simulink model "PREPROCESS"  (R2020b)
settings: Solver=FixedStepAuto  StartTime=0.0  StopTime=31622400  FixedStep=60  RelTol=1e-3
libraries: simulink x30
(part 1 of 2)
settings Model: Creator=khfa  LastModifiedBy=khfa

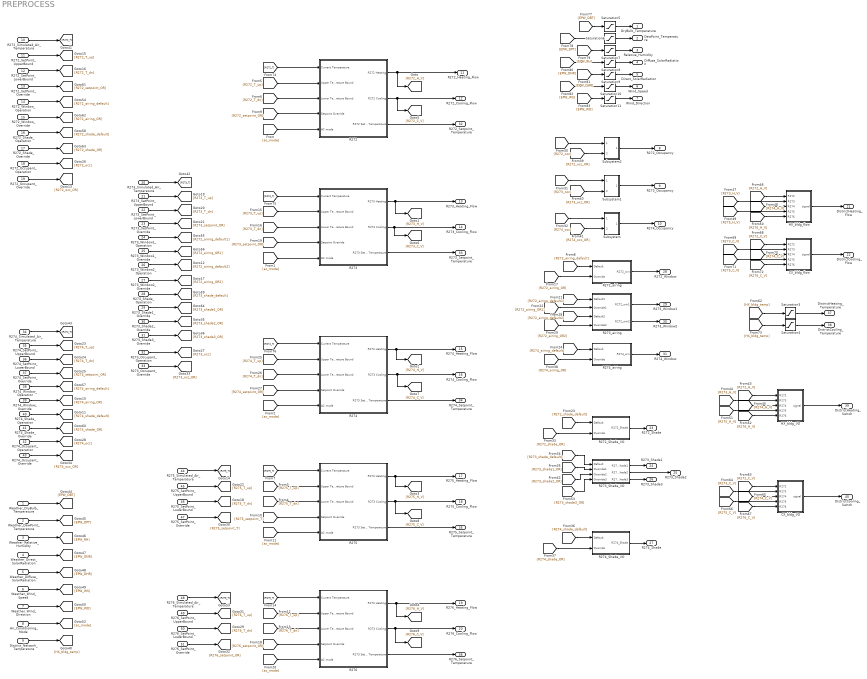
== system PREPROCESS ==
  Weather_DryBulb_Temperature : Inport
  Weather_DewPoint_Temperature : Inport  Port=2
  Weather_Relative_Humidity : Inport  Port=3
  Weather_Direct_SolarRadiation : Inport  Port=4
  Weather_Diffuse_SolarRadiation : Inport  Port=5
  Weather_Wind_Speed : Inport  Port=6
  Weather_Wind_Direction : Inport  Port=7
  Air_Conditioning_Mode : Inport  Port=8
  District_Network_Temperature : Inport  Port=9
  R272_Simulated_Air_Temperature : Inport  Port=10  SampleTime=60
  R272_SetPoint_UpperBound : Inport  Port=11
  R272_SetPoint_LowerBound : Inport  Port=12
  R272_SetPoint_Override : Inport  Port=13
  R272_Window_Operation : Inport  Port=14
  R272_Window_Override : Inport  Port=15
  R272_Shade_Operation : Inport  Port=16
  R272_Shade_Override : Inport  Port=17
  R272_Occupant_Operation : Inport  Port=18
  R272_Occupant_Override : Inport  Port=19
  R273_Simulated_Air_Temperature : Inport  Port=20  SampleTime=60
  R273_SetPoint_UpperBound : Inport  Port=21
  R273_SetPoint_LowerBound : Inport  Port=22
  R273_SetPoint_Override : Inport  Port=23
  R273_Window1_Operation : Inport  Port=24
  R273_Window1_Override : Inport  Port=25
  R273_Window2_Operation : Inport  Port=26
  R273_Window2_Override : Inport  Port=27
  R273_Shade_Operation : Inport  Port=28
  R273_Shade1_Override : Inport  Port=29
  R273_Shade2_Override : Inport  Port=30
  R273_Shade3_Override : Inport  Port=31
  R273_Occupant_Operation : Inport  Port=32
  R273_Occupant_Override : Inport  Port=33
  R274_Simulated_Air_Temperature : Inport  Port=34  SampleTime=60
  R274_SetPoint_UpperBound : Inport  Port=35
  R274_SetPoint_LowerBound : Inport  Port=36
  R274_SetPoint_Override : Inport  Port=37
  R274_Window_Operation : Inport  Port=38
  R274_Window_Override : Inport  Port=39
  R274_Shade_Operation : Inport  Port=40
  R274_Shade_Override : Inport  Port=41
  R274_Occupant_Operation : Inport  Port=42
  R274_Occupant_Override : Inport  Port=43
  R275_Simulated_Air_Temperature : Inport  Port=44  SampleTime=60
  R275_SetPoint_UpperBound : Inport  Port=45
  R275_SetPoint_LowerBound : Inport  Port=46
  R275_SetPoint_Override : Inport  Port=47
  R276_Simulated_Air_Temperature : Inport  Port=48  SampleTime=60
  R276_SetPoint_UpperBound : Inport  Port=49
  R276_SetPoint_LowerBound : Inport  Port=50
  R276_SetPoint_Override : Inport  Port=51
  CX_bldg_I/O : Subsystem
  CX_bldg_flow : Subsystem
  HX_bldg_I/O : Subsystem
  HX_bldg_flow : Subsystem
  R272 : Subsystem
  R272_Shade_I/O : Subsystem
  R272_airing : Subsystem
  R273 : Subsystem
  R273_Shade_I/O : Subsystem
  R273_airing : Subsystem
  R274 : Subsystem
  R274_Shade_I/O : Subsystem
  R274_airing : Subsystem
  R275 : Subsystem
  R276 : Subsystem
  Saturation10 : Saturate  UpperLimit=50  LowerLimit=0
  Saturation11 : Saturate  UpperLimit=360  LowerLimit=0
  Saturation3 : Saturate  UpperLimit=60  LowerLimit=20
  Saturation4 : Saturate  UpperLimit=40  LowerLimit=0
  Saturation5 : Saturate  UpperLimit=60  LowerLimit=-60
  Saturation6 : Saturate  UpperLimit=60  LowerLimit=-60
  Saturation7 : Saturate  UpperLimit=100  LowerLimit=0
  Saturation8 : Saturate  UpperLimit=1000  LowerLimit=0
  Saturation9 : Saturate  UpperLimit=1500  LowerLimit=0
  Subsystem : Subsystem
  Subsystem1 : Subsystem
  Subsystem2 : Subsystem
  DryBulb_Temperature : Outport
  DewPoint_Temperature : Outport  Port=2
  Relative_Humidity : Outport  Port=3
  Diffuse_SolarRadiation : Outport  Port=4
  Direct_SolarRadiation : Outport  Port=5
  Wind_Speed : Outport  Port=6
  Wind_Direction : Outport  Port=7
  R272_Occupancy : Outport  Port=8
  R273_Occupancy : Outport  Port=9
  R274_Occupancy : Outport  Port=10
  R272_Heating_Flow : Outport  Port=11
  R272_Cooling_Flow : Outport  Port=12
  R273_Heating_Flow : Outport  Port=13
  R273_Cooling_Flow : Outport  Port=14
  R274_Heating_Flow : Outport  Port=15
  R274_Cooling_Flow : Outport  Port=16
  R275_Heating_Flow : Outport  Port=17
  R275_Cooling_Flow : Outport  Port=18
  R276_Heating_Flow : Outport  Port=19
  R276_Cooling_Flow : Outport  Port=20
  DistrictHeating_Flow : Outport  Port=21
  DistrictCooling_Flow : Outport  Port=22
  R272_Shade : Outport  Port=23
  R273_Shade1 : Outport  Port=24
  R273_Shade2 : Outport  Port=25
  R273_Shade3 : Outport  Port=26
  R274_Shade : Outport  Port=27
  R272_Window : Outport  Port=28
  R273_Window1 : Outport  Port=29
  R273_Window2 : Outport  Port=30
  R274_Window : Outport  Port=31
  R272_Setpoint_Temperature : Outport  Port=32
  R273_Setpoint_Temperature : Outport  Port=33
  R274_Setpoint_Temperature : Outport  Port=34
  R275_Setpoint_Temperature : Outport  Port=35
  R276_Setpoint_Temperature : Outport  Port=36
  DistrictHeating_Temperature : Outport  Port=37
  DistrictCooling_Temperature : Outport  Port=38
  DistrictHeating_Switch : Outport  Port=39
  DistrictCooling_Switch : Outport  Port=40
  wires:
  Saturation11/1 -> Wind_Direction/1
  Saturation6/1 -> DewPoint_Temperature/1
  Saturation7/1 -> Relative_Humidity/1
  Saturation8/1 -> Diffuse_SolarRadiation/1
  Saturation10/1 -> Wind_Speed/1
  R272_Shade_I/O/1(R272_Shade) -> R272_Shade/1
  R273_Shade_I/O/1(R273_Shade1) -> R273_Shade1/1
  R275_Simulated_Air_Temperature/1 -> [R275_T]
  R275_SetPoint_Override/1 -> [R275_setpoint_T]
  R275_SetPoint_LowerBound/1 -> [R275_T_dn]
  R274/3(R273 Setpoint Temperature) -> R274_Setpoint_Temperature/1
  R275/3(R273 Setpoint Temperature) -> R275_Setpoint_Temperature/1
  R273_Window2_Operation/1 -> [R272_airing_default2]
  District_Network_Temperature/1 -> [HX_bldg_temp]
  Weather_Direct_SolarRadiation/1 -> [EPW_DNR]
  R273/3(R273 Setpoint Temperature) -> R273_Setpoint_Temperature/1
  Weather_Wind_Speed/1 -> [EPW_WS]
  R273_Occupant_Operation/1 -> [R273_occ]
  R273_SetPoint_LowerBound/1 -> [R273_T_dn]
  R273_Simulated_Air_Temperature/1 -> [R273_T]
  R273_SetPoint_Override/1 -> [R273_setpoint_OR]
  Air_Conditioning_Mode/1 -> [ac_mode]
  R273_Window1_Operation/1 -> [R272_airing_default1]
  R273_SetPoint_UpperBound/1 -> [R273_T_up]
  R273_Shade_Operation/1 -> [R273_shade_default]
  R273_Window1_Override/1 -> [R272_airing_OR1]
  R273_Shade1_Override/1 -> [R273_shade1_OR]
  R273_Window2_Override/1 -> [R272_airing_OR2]
  Weather_Relative_Humidity/1 -> [EPW_RH]
  Weather_Diffuse_SolarRadiation/1 -> [EPW_DHR]
  Weather_Wind_Direction/1 -> [EPW_WD]
  CX_bldg_I/O/1(signal) -> DistrictCooling_Switch/1
  Saturation4/1 -> DistrictCooling_Temperature/1
  HX_bldg_I/O/1(signal) -> DistrictHeating_Switch/1
  Saturation3/1 -> DistrictHeating_Temperature/1
  R272_SetPoint_UpperBound/1 -> [R272_T_up]
  R272_Window_Operation/1 -> [R272_airing_default]
  R272_Occupant_Operation/1 -> [R272_occ]
  R272_Shade_Operation/1 -> [R272_shade_default]
  R272_Window_Override/1 -> [R272_airing_OR]
  R272_SetPoint_Override/1 -> [R272_setpoint_OR]
  [R276_C_V] -> CX_bldg_I/O/5(R276)
  [R275_C_V] -> CX_bldg_flow/4(R275)
  [R272_H_V] -> HX_bldg_I/O/1(R272)
  R272_SetPoint_LowerBound/1 -> [R272_T_dn]
  [R272_setpoint_OR] -> R272/4(Setpoint Override)
  Saturation5/1 -> DryBulb_Temperature/1
  [R272_T] -> R272/1(Current Temperature)
  [R274_C_V] -> CX_bldg_I/O/3(R274)
  [R275_H_V] -> HX_bldg_I/O/4(R275)
  R272/3(R272 Setpoint Temperature) -> R272_Setpoint_Temperature/1
  [R273_H_V] -> HX_bldg_I/O/2(R273)
  [R276_H_V] -> HX_bldg_I/O/5(R276)
  [R272_H_V] -> HX_bldg_flow/1(R272)
  [R276_T_up] -> R276/2(Upper Temperature Bound)
  [R273_T_up] -> R273/2(Upper Temperature Bound)
  [R275_T_up] -> R275/2(Upper Temperature Bound)
  Saturation9/1 -> Direct_SolarRadiation/1
  [EPW_DPT] -> Saturation6/1
  [R272_airing_default] -> R272_airing/1(Default)
  R273/2(R273 Cooling) -> R273_Cooling_Flow/1, [R273_C_V]
  R272/1(R272 Heating) -> R272_Heating_Flow/1, [R272_H_V]
  R274/1(R273 Heating) -> R274_Heating_Flow/1, [R274_H_V]
  R275/1(R273 Heating) -> R275_Heating_Flow/1, [R275_H_V]
  [R275_T] -> R275/1(Current Temperature)
  [R273_setpoint_OR] -> R273/4(Setpoint Override)
  [R276_C_V] -> CX_bldg_flow/5(R276)
  R272_Simulated_Air_Temperature/1 -> [R272_T]
  [R273_C_V] -> CX_bldg_flow/2(R273)
  [EPW_DHR] -> Saturation9/1
  [R274_T_dn] -> R274/3(Lower Temperature Bound)
  R272/2(R272 Cooling) -> R272_Cooling_Flow/1, [R272_C_V]
  R272_Shade_Override/1 -> [R272_shade_OR]
  [R273_T_dn] -> R273/3(Lower Temperature Bound)
  R273/1(R273 Heating) -> [R273_H_V], R273_Heating_Flow/1
  [EPW_RH] -> Saturation7/1
  [ac_mode] -> R272/5(AC mode)
  [EPW_DBT] -> Saturation5/1
  [R274_T_up] -> R274/2(Upper Temperature Bound)
  [R272_C_V] -> CX_bldg_I/O/1(R272)
  [HX_bldg_temp] -> Saturation3/1
  [R274_shade_OR] -> R274_Shade_I/O/2(Override)
  Weather_DewPoint_Temperature/1 -> [EPW_DPT]
  [HX_bldg_temp] -> Saturation4/1
  [R273_shade1_OR] -> R273_Shade_I/O/2(Override1)
  [R273_shade_default] -> R273_Shade_I/O/1(Default)
  [R274_H_V] -> HX_bldg_I/O/3(R274)
  R276_SetPoint_LowerBound/1 -> [R276_T_dn]
  R276_Simulated_Air_Temperature/1 -> [R276_T]
  CX_bldg_flow/1(signal) -> DistrictCooling_Flow/1
  [R272_airing_default1] -> R273_airing/1(Default1)
  R276/1(R273 Heating) -> R276_Heating_Flow/1, [R276_H_V]
  R274_SetPoint_UpperBound/1 -> [R274_T_up]
  R274_SetPoint_LowerBound/1 -> [R274_T_dn]
  R276_SetPoint_Override/1 -> [R276_setpoint_OR]
  [EPW_WD] -> Saturation11/1
  [R274_airing_OR] -> R274_airing/2(Override)
  HX_bldg_flow/1(signal) -> DistrictHeating_Flow/1
  [R273_T] -> R273/1(Current Temperature)
  [R272_airing_default2] -> R273_airing/3(Default2)
  [R272_shade_OR] -> R272_Shade_I/O/2(Override)
  [R272_airing_OR2] -> R273_airing/4(Override2)
  R274_Shade_Override/1 -> [R274_shade_OR]
  [R272_airing_OR1] -> R273_airing/2(Override1)
  [R272_shade_default] -> R272_Shade_I/O/1(Default)
  [R274_H_V] -> HX_bldg_flow/3(R274)
  [R272_C_V] -> CX_bldg_flow/1(R272)
  R275_SetPoint_UpperBound/1 -> [R275_T_up]
  R276/2(R273 Cooling) -> R276_Cooling_Flow/1, [R276_C_V]
  [EPW_WS] -> Saturation10/1
  [R274_C_V] -> CX_bldg_flow/3(R274)
  [R273_C_V] -> CX_bldg_I/O/2(R273)
  [R275_T_dn] -> R275/3(Lower Temperature Bound)
  [ac_mode] -> R275/5(AC mode)
  [R272_T_dn] -> R272/3(Lower Temperature Bound)
  R274_Window_Operation/1 -> [R274_airing_default]
  [R276_setpoint_OR] -> R276/4(Setpoint Override)
  [R275_setpoint_T] -> R275/4(Setpoint Override)
  [R275_C_V] -> CX_bldg_I/O/4(R275)
  [R272_airing_OR] -> R272_airing/2(Override)
  R274_Simulated_Air_Temperature/1 -> [R274_T]
  R274/2(R273 Cooling) -> R274_Cooling_Flow/1, [R274_C_V]
  [R275_H_V] -> HX_bldg_flow/4(R275)
  R276_SetPoint_UpperBound/1 -> [R276_T_up]
  [R274_shade_default] -> R274_Shade_I/O/1(Default)
  [R274_T] -> R274/1(Current Temperature)
  R275/2(R273 Cooling) -> [R275_C_V], R275_Cooling_Flow/1
  R274_Shade_Operation/1 -> [R274_shade_default]
  [R272_T_up] -> R272/2(Upper Temperature Bound)
  R274_Shade_I/O/1(R274_Shade) -> R274_Shade/1
  [ac_mode] -> R276/5(AC mode)
  [R274_airing_default] -> R274_airing/1(Default)
  R274_Window_Override/1 -> [R274_airing_OR]
  [ac_mode] -> R273/5(AC mode)
  Weather_DryBulb_Temperature/1 -> [EPW_DBT]
  [R276_T_dn] -> R276/3(Lower Temperature Bound)
  R273_airing/1(R272_win1) -> R273_Window1/1
  [EPW_DNR] -> Saturation8/1
  R274_SetPoint_Override/1 -> [R274_setpoint_OR]
  R272_airing/1(R272_win) -> R272_Window/1
  R274_airing/1(R274_win) -> R274_Window/1
  [R273_H_V] -> HX_bldg_flow/2(R273)
  [R274_setpoint_OR] -> R274/4(Setpoint Override)
  [R276_T] -> R276/1(Current Temperature)
  R274_Occupant_Operation/1 -> [R274_occ]
  R273_airing/2(R272_win2) -> R273_Window2/1
  R276/3(R273 Setpoint Temperature) -> R276_Setpoint_Temperature/1
  [R276_H_V] -> HX_bldg_flow/5(R276)
  [ac_mode] -> R274/5(AC mode)
  R272_Occupant_Override/1 -> [R272_occ_OR]
  R273_Occupant_Override/1 -> [R273_occ_OR]
  R274_Occupant_Override/1 -> [R274_occ_OR]
  [R274_occ] -> Subsystem/1(In1)
  [R274_occ_OR] -> Subsystem/2(In2)
  Subsystem/1(Out1) -> R274_Occupancy/1
  [R273_occ] -> Subsystem1/1(In1)
  [R273_occ_OR] -> Subsystem1/2(In2)
  Subsystem1/1(Out1) -> R273_Occupancy/1
  [R272_occ] -> Subsystem2/1(In1)
  [R272_occ_OR] -> Subsystem2/2(In2)
  Subsystem2/1(Out1) -> R272_Occupancy/1
  R273_Shade2_Override/1 -> [R273_shade2_OR]
  R273_Shade3_Override/1 -> [R273_shade3_OR]
  R273_Shade_I/O/2(R273_Shade2) -> R273_Shade2/1
  R273_Shade_I/O/3(R273_Shade3) -> R273_Shade3/1
  [R273_shade2_OR] -> R273_Shade_I/O/3(Override2)
  [R273_shade3_OR] -> R273_Shade_I/O/4(Override3)

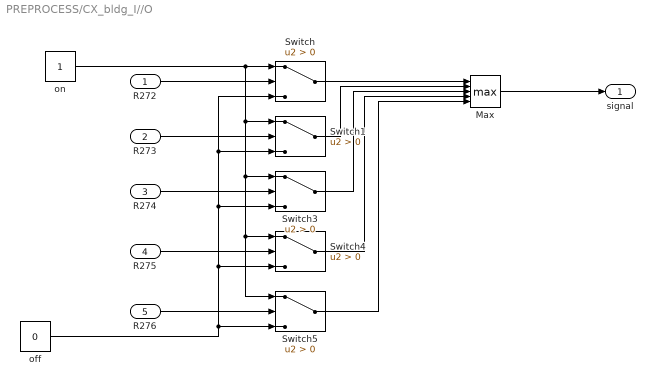
== system PREPROCESS/CX_bldg_I//O ==
  R272 : Inport
  R273 : Inport  Port=2
  R274 : Inport  Port=3
  R275 : Inport  Port=4
  R276 : Inport  Port=5
  Max : MinMax  Function=max  Inputs=5
  Switch{,1,3..5} (5 alike) : Switch  Criteria=u2 > Threshold
  off : Constant  Value=0
  on : Constant
  signal : Outport
  wires:
  on/1 -> Switch5/1, Switch4/1, Switch3/1, Switch1/1, Switch/1
  R272/1 -> Switch/2
  off/1 -> Switch5/3, Switch3/3, Switch1/3, Switch/3, Switch4/3
  R273/1 -> Switch1/2
  R274/1 -> Switch3/2
  Switch/1 -> Max/1
  Switch1/1 -> Max/2
  Switch3/1 -> Max/3
  R276/1 -> Switch5/2
  R275/1 -> Switch4/2
  Switch4/1 -> Max/4
  Switch5/1 -> Max/5
  Max/1 -> signal/1

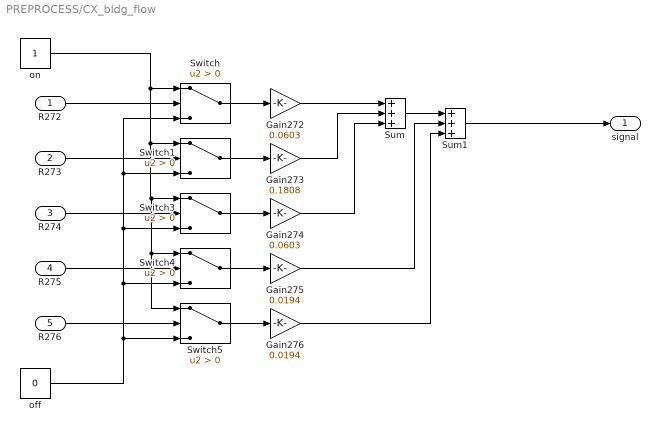
== system PREPROCESS/CX_bldg_flow ==
  R272 : Inport
  R273 : Inport  Port=2
  R274 : Inport  Port=3
  R275 : Inport  Port=4
  R276 : Inport  Port=5
  Gain272 : Gain  Gain=0.0603
  Gain273 : Gain  Gain=0.1808
  Gain274 : Gain  Gain=0.0603
  Gain275 : Gain  Gain=0.0194
  Gain276 : Gain  Gain=0.0194
  Sum : Sum  Inputs=+++
  Sum1 : Sum  Inputs=+++
  Switch{,1,3..5} (5 alike) : Switch  Criteria=u2 > Threshold
  off : Constant  Value=0
  on : Constant
  signal : Outport
  wires:
  Sum/1 -> Sum1/1
  on/1 -> Switch5/1, Switch4/1, Switch3/1, Switch1/1, Switch/1
  R272/1 -> Switch/2
  off/1 -> Switch4/3, Switch3/3, Switch1/3, Switch/3, Switch5/3
  R273/1 -> Switch1/2
  R274/1 -> Switch3/2
  Switch/1 -> Gain272/1
  Switch1/1 -> Gain273/1
  Switch3/1 -> Gain274/1
  Gain272/1 -> Sum/1
  Gain274/1 -> Sum/3
  Gain273/1 -> Sum/2
  Switch4/1 -> Gain275/1
  Gain275/1 -> Sum1/2
  Switch5/1 -> Gain276/1
  R275/1 -> Switch4/2
  R276/1 -> Switch5/2
  Gain276/1 -> Sum1/3
  Sum1/1 -> signal/1

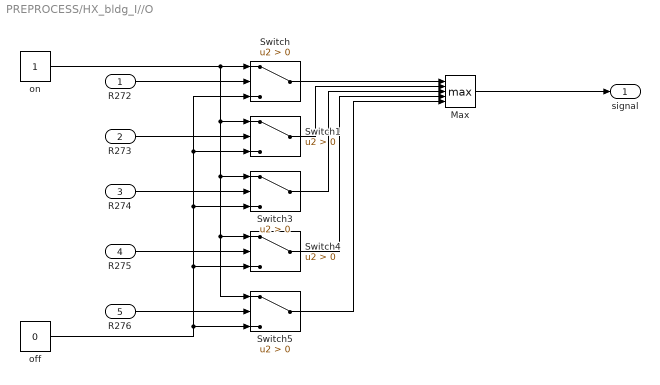
== system PREPROCESS/HX_bldg_I//O ==
  R272 : Inport
  R273 : Inport  Port=2
  R274 : Inport  Port=3
  R275 : Inport  Port=4
  R276 : Inport  Port=5
  Max : MinMax  Function=max  Inputs=5
  Switch{,1,3..5} (5 alike) : Switch  Criteria=u2 > Threshold
  off : Constant  Value=0
  on : Constant
  signal : Outport
  wires:
  Max/1 -> signal/1
  on/1 -> Switch5/1, Switch4/1, Switch3/1, Switch1/1, Switch/1
  R272/1 -> Switch/2
  off/1 -> Switch5/3, Switch3/3, Switch1/3, Switch/3, Switch4/3
  R273/1 -> Switch1/2
  R274/1 -> Switch3/2
  Switch/1 -> Max/1
  Switch1/1 -> Max/2
  Switch3/1 -> Max/3
  R276/1 -> Switch5/2
  R275/1 -> Switch4/2
  Switch4/1 -> Max/4
  Switch5/1 -> Max/5

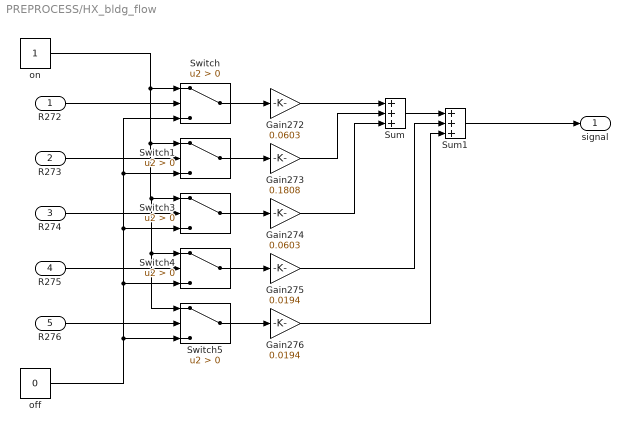
== system PREPROCESS/HX_bldg_flow ==
  R272 : Inport
  R273 : Inport  Port=2
  R274 : Inport  Port=3
  R275 : Inport  Port=4
  R276 : Inport  Port=5
  Gain272 : Gain  Gain=0.0603
  Gain273 : Gain  Gain=0.1808
  Gain274 : Gain  Gain=0.0603
  Gain275 : Gain  Gain=0.0194
  Gain276 : Gain  Gain=0.0194
  Sum : Sum  Inputs=+++
  Sum1 : Sum  Inputs=+++
  Switch{,1,3..5} (5 alike) : Switch  Criteria=u2 > Threshold
  off : Constant  Value=0
  on : Constant
  signal : Outport
  wires:
  Sum/1 -> Sum1/1
  on/1 -> Switch5/1, Switch4/1, Switch3/1, Switch1/1, Switch/1
  R272/1 -> Switch/2
  off/1 -> Switch4/3, Switch3/3, Switch1/3, Switch/3, Switch5/3
  R273/1 -> Switch1/2
  R274/1 -> Switch3/2
  Switch/1 -> Gain272/1
  Switch1/1 -> Gain273/1
  Switch3/1 -> Gain274/1
  Gain272/1 -> Sum/1
  Gain274/1 -> Sum/3
  Gain273/1 -> Sum/2
  Switch4/1 -> Gain275/1
  Gain275/1 -> Sum1/2
  Switch5/1 -> Gain276/1
  R275/1 -> Switch4/2
  R276/1 -> Switch5/2
  Gain276/1 -> Sum1/3
  Sum1/1 -> signal/1

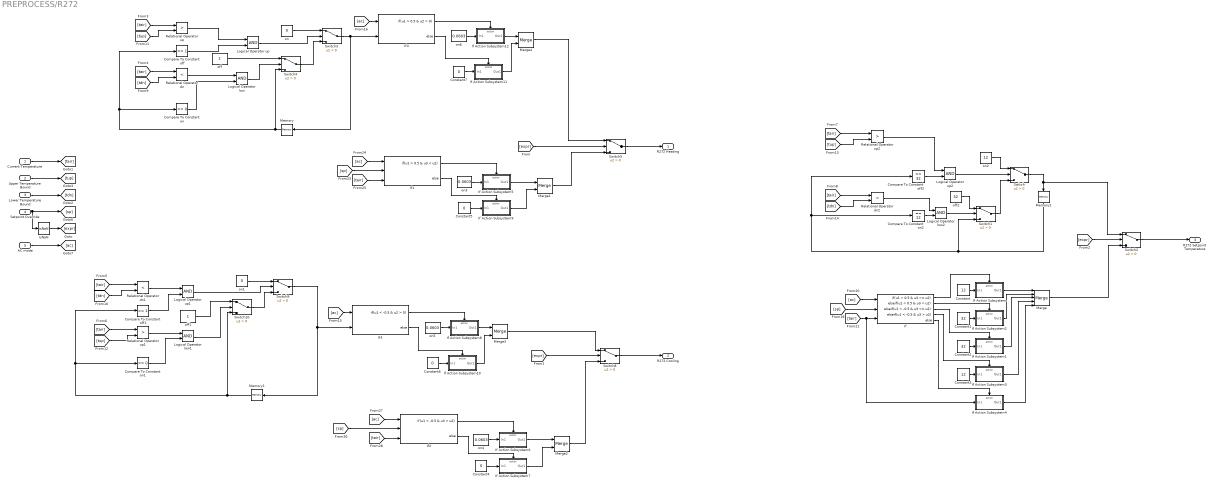
== system PREPROCESS/R272 ==
  Current Temperature : Inport
  Upper Temperature Bound : Inport  Port=2
  Lower Temperature Bound : Inport  Port=3
  Setpoint Override : Inport  Port=4
  AC mode : Inport  Port=5
  Compare To Constant off : simulink/Logic and Bit Operations/Compare To Constant  relop===  const=1  OutDataTypeStr=boolean
  Compare To Constant off1 : simulink/Logic and Bit Operations/Compare To Constant  relop===  const=1  OutDataTypeStr=boolean
  Compare To Constant off2 : simulink/Logic and Bit Operations/Compare To Constant  relop===  const=32  OutDataTypeStr=boolean
  Compare To Constant on : simulink/Logic and Bit Operations/Compare To Constant  relop===  const=0  OutDataTypeStr=boolean
  Compare To Constant on1 : simulink/Logic and Bit Operations/Compare To Constant  relop===  const=0  OutDataTypeStr=boolean
  Compare To Constant on2 : simulink/Logic and Bit Operations/Compare To Constant  relop===  const=12  OutDataTypeStr=boolean
  Constant : Constant  Value=12
  Constant1 : Constant  Value=32
  Constant2 : Constant  Value=32
  Constant3 : Constant  Value=12
  Constant{4..7} (4 alike) : Constant  Value=0
  If : If  NumInputs=3  IfExpression=u1 > 0.5 & u3 >= u2  ElseIfExpressions=u1 > 0.5 & u3 < u2, u1 < -0.5 & u3 <= u2, u1 < -0.5 & u3 > u2
  If Action Subsystem : Subsystem  TreatAsAtomicUnit=on
  If Action Subsystem1 : Subsystem  TreatAsAtomicUnit=on
  If Action Subsystem10 : Subsystem  TreatAsAtomicUnit=on
  If Action Subsystem11 : Subsystem  TreatAsAtomicUnit=on
  If Action Subsystem12 : Subsystem  TreatAsAtomicUnit=on
  If Action Subsystem2 : Subsystem  TreatAsAtomicUnit=on
  If Action Subsystem3 : Subsystem  TreatAsAtomicUnit=on
  If Action Subsystem4 : Subsystem  TreatAsAtomicUnit=on
  If Action Subsystem5 : Subsystem  TreatAsAtomicUnit=on
  If Action Subsystem6 : Subsystem  TreatAsAtomicUnit=on
  If Action Subsystem7 : Subsystem  TreatAsAtomicUnit=on
  If Action Subsystem8 : Subsystem  TreatAsAtomicUnit=on
  If Action Subsystem9 : Subsystem  TreatAsAtomicUnit=on
  If1 : If  NumInputs=3  IfExpression=u1 > 0.5 & u3 < u2
  If2 : If  NumInputs=3  IfExpression=u1 < -0.5 & u3 > u2
  If3 : If  NumInputs=2  IfExpression=u1 < -0.5 & u2 > 0
  If4 : If  NumInputs=2  IfExpression=u1 > 0.5 & u2 > 0
  IsNaN : RelationalOperator  Operator=isNaN  OutDataTypeStr=boolean  RndMeth=Simplest
  Logical Operator low : Logic  AllPortsSameDT=off  OutDataTypeStr=boolean
  Logical Operator low1 : Logic  AllPortsSameDT=off  OutDataTypeStr=boolean
  Logical Operator low2 : Logic  AllPortsSameDT=off  OutDataTypeStr=boolean
  Logical Operator up : Logic  AllPortsSameDT=off  OutDataTypeStr=boolean
  Logical Operator up1 : Logic  AllPortsSameDT=off  OutDataTypeStr=boolean
  Logical Operator up2 : Logic  AllPortsSameDT=off  OutDataTypeStr=boolean
  Memory : Memory
  Memory1 : Memory
  Memory2 : Memory  InitialCondition=12
  Merge : Merge  Inputs=5
  Merge{1..4} (4 alike) : Merge
  Relational Operator dn : RelationalOperator  Operator=<  OutDataTypeStr=boolean  RndMeth=Simplest
  Relational Operator dn1 : RelationalOperator  Operator=<  OutDataTypeStr=boolean  RndMeth=Simplest
  Relational Operator dn2 : RelationalOperator  Operator=<  OutDataTypeStr=boolean  RndMeth=Simplest
  Relational Operator up : RelationalOperator  Operator=>  OutDataTypeStr=boolean  RndMeth=Simplest
  Relational Operator up1 : RelationalOperator  Operator=>  OutDataTypeStr=boolean  RndMeth=Simplest
  Relational Operator up2 : RelationalOperator  Operator=>  OutDataTypeStr=boolean  RndMeth=Simplest
  Switch{,1..5,8..10} (9 alike) : Switch  Criteria=u2 > Threshold
  off : Constant
  off1 : Constant
  off2 : Constant  Value=32
  on : Constant  Value=0
  on1 : Constant  Value=0
  on2 : Constant  Value=12
  on{3..6} (4 alike) : Constant  Value=0.0603
  R272 Heating : Outport
  R272 Cooling : Outport  Port=2
  R272 Setpoint Temperature : Outport  Port=3
  wires:
  [tup] -> Relational Operator up2/2
  [tdn] -> Relational Operator dn2/2
  If4/1 -> If Action Subsystem12/Action
  If4/2 -> If Action Subsystem11/Action
  IsNaN/1 -> [expr]
  If Action Subsystem11/1(Out1) -> Merge4/2
  If/4 -> If Action Subsystem3/Action
  on2/1 -> Switch/1
  [tair] -> If1/3
  If Action Subsystem10/1(Out1) -> Merge3/2
  on6/1 -> If Action Subsystem12/1(In1)
  Merge2/1 -> Switch8/3
  Constant7/1 -> If Action Subsystem11/1(In1)
  [expr] -> Switch5/2
  If1/2 -> If Action Subsystem9/Action
  [sp] -> If/2
  [tup] -> Relational Operator up/2
  Relational Operator dn/1 -> Logical Operator low/1
  [tair] -> If Action Subsystem4/1(In1), If/3
  If Action Subsystem3/1(Out1) -> Merge/4
  If2/1 -> If Action Subsystem6/Action
  If3/1 -> If Action Subsystem8/Action
  If1/1 -> If Action Subsystem5/Action
  [ac] -> If3/1
  Merge4/1 -> Switch5/1
  If2/2 -> If Action Subsystem7/Action
  Compare To Constant off/1 -> Logical Operator up/2
  If Action Subsystem4/1(Out1) -> Merge/5
  Constant2/1 -> If Action Subsystem1/1(In1)
  Lower Temperature Bound/1 -> [tdn]
  Constant6/1 -> If Action Subsystem10/1(In1)
  Relational Operator up2/1 -> Logical Operator up2/1
  on5/1 -> If Action Subsystem8/1(In1)
  Compare To Constant on/1 -> Logical Operator low/2
  Switch5/1 -> R272 Heating/1
  If3/2 -> If Action Subsystem10/Action
  Switch9/1 -> If3/2, Memory1/1
  Switch4/1 -> Switch3/3
  [sp] -> If2/2
  [ac] -> If4/1
  If/5 -> If Action Subsystem4/Action
  on4/1 -> If Action Subsystem6/1(In1)
  Switch8/1 -> R272 Cooling/1
  If Action Subsystem8/1(Out1) -> Merge3/1
  [sp] -> If1/2
  Constant4/1 -> If Action Subsystem7/1(In1)
  Memory/1 -> Compare To Constant on/1, Compare To Constant off/1, Switch4/3
  If Action Subsystem7/1(Out1) -> Merge2/2
  If Action Subsystem6/1(Out1) -> Merge2/1
  Merge3/1 -> Switch8/1
  Logical Operator up/1 -> Switch3/2
  AC mode/1 -> [ac]
  Constant1/1 -> If Action Subsystem2/1(In1)
  Switch3/1 -> Memory/1, If4/2
  [tair] -> If2/3
  If Action Subsystem1/1(Out1) -> Merge/3
  If Action Subsystem5/1(Out1) -> Merge1/1
  If Action Subsystem/1(Out1) -> Merge/1
  If Action Subsystem9/1(Out1) -> Merge1/2
  Merge1/1 -> Switch5/3
  on3/1 -> If Action Subsystem5/1(In1)
  If/2 -> If Action Subsystem2/Action
  Setpoint Override/1 -> IsNaN/1, [sp]
  [ac] -> If2/1
  off1/1 -> Switch10/1
  [tair] -> Relational Operator up2/1
  If/3 -> If Action Subsystem1/Action
  Logical Operator low1/1 -> Switch10/2
  Compare To Constant on1/1 -> Logical Operator low1/2
  Compare To Constant off2/1 -> Logical Operator up2/2
  [tair] -> Relational Operator dn2/1
  [tair] -> Relational Operator up1/1
  [tair] -> Relational Operator dn1/1
  If/1 -> If Action Subsystem/Action
  Constant/1 -> If Action Subsystem/1(In1)
  Logical Operator up2/1 -> Switch/2
  Constant3/1 -> If Action Subsystem3/1(In1)
  Logical Operator low2/1 -> Switch1/2
  Compare To Constant on2/1 -> Logical Operator low2/2
  Memory2/1 -> Compare To Constant on2/1, Compare To Constant off2/1, Switch1/3
  off2/1 -> Switch1/1
  Switch1/1 -> Switch/3
  Switch2/1 -> R272 Setpoint Temperature/1
  [ac] -> If1/1
  [tair] -> Relational Operator dn/1
  [expr] -> Switch8/2
  [tair] -> Relational Operator up/1
  If Action Subsystem12/1(Out1) -> Merge4/1
  Relational Operator dn2/1 -> Logical Operator low2/1
  Logical Operator low/1 -> Switch4/2
  Upper Temperature Bound/1 -> [tup]
  Compare To Constant off1/1 -> Logical Operator up1/2
  Merge/1 -> Switch2/3
  Memory1/1 -> Compare To Constant on1/1, Compare To Constant off1/1, Switch10/3
  [tup] -> Relational Operator up1/2
  [tdn] -> Relational Operator dn1/2
  Relational Operator up1/1 -> Logical Operator low1/1
  Relational Operator dn1/1 -> Logical Operator up1/1
  off/1 -> Switch4/1
  [ac] -> If/1
  Switch10/1 -> Switch9/3
  [tdn] -> Relational Operator dn/2
  Constant5/1 -> If Action Subsystem9/1(In1)
  Relational Operator up/1 -> Logical Operator up/1
  on/1 -> Switch3/1
  [expr] -> Switch2/2
  If Action Subsystem2/1(Out1) -> Merge/2
  Logical Operator up1/1 -> Switch9/2
  Current Temperature/1 -> [tair]
  Switch/1 -> Switch2/1, Memory2/1
  on1/1 -> Switch9/1

== system PREPROCESS/R272_Shade_I//O ==
  Default : Inport
  Override : Inport  Port=2
  Constant : Constant
  Constant1 : Constant  Value=0
  IsNaN : RelationalOperator  Operator=isNaN  OutDataTypeStr=boolean  RndMeth=Simplest
  R272_lum_limit : Switch  Criteria=u2 > Threshold  Threshold=50
  Switch : Switch  Criteria=u2 > Threshold
  Switch1 : Switch  Criteria=u2 > Threshold
  off1 : Constant
  on1 : Constant  Value=0
  R272_Shade : Outport
  wires:
  off1/1 -> R272_lum_limit/3
  on1/1 -> R272_lum_limit/1
  Default/1 -> R272_lum_limit/2
  Constant/1 -> Switch/1
  Constant1/1 -> Switch/3
  Override/1 -> IsNaN/1, Switch/2
  R272_lum_limit/1 -> Switch1/1
  Switch1/1 -> R272_Shade/1
  Switch/1 -> Switch1/3
  IsNaN/1 -> Switch1/2

== system PREPROCESS/R272_airing ==
  Default : Inport
  Override : Inport  Port=2
  Constant : Constant  Value=-49
  Constant1 : Constant  Value=99
  IsNaN : RelationalOperator  Operator=isNaN  OutDataTypeStr=boolean  RndMeth=Simplest
  Switch : Switch  Criteria=u2 > Threshold
  Switch1 : Switch  Criteria=u2 > Threshold
  R272_win : Outport
  wires:
  Constant/1 -> Switch/1
  Constant1/1 -> Switch/3
  Override/1 -> IsNaN/1, Switch/2
  Switch/1 -> Switch1/3
  Switch1/1 -> R272_win/1
  Default/1 -> Switch1/1
  IsNaN/1 -> Switch1/2

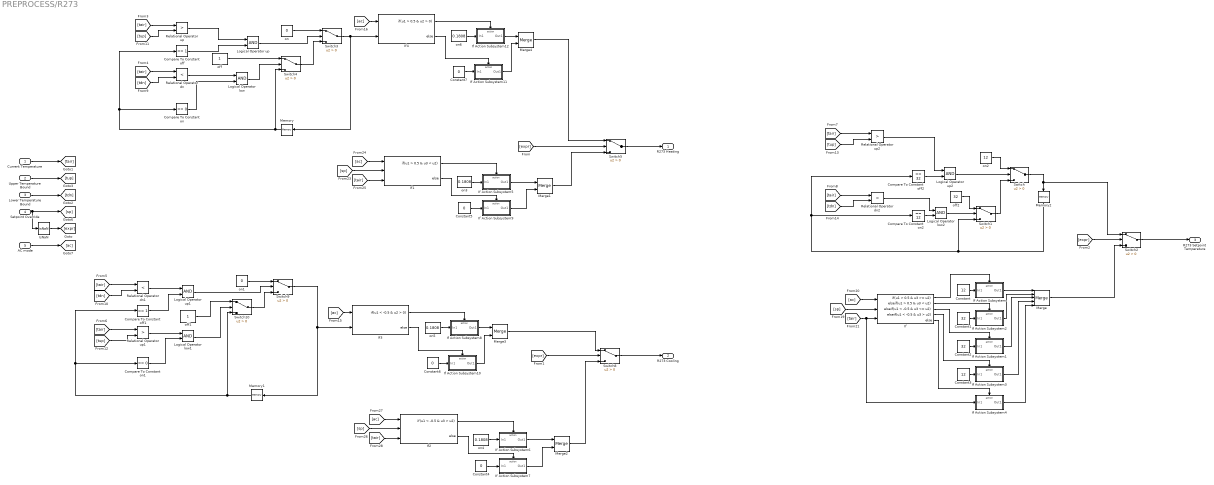
== system PREPROCESS/R273 ==
  Current Temperature : Inport
  Upper Temperature Bound : Inport  Port=2
  Lower Temperature Bound : Inport  Port=3
  Setpoint Override : Inport  Port=4
  AC mode : Inport  Port=5
  Compare To Constant off : simulink/Logic and Bit Operations/Compare To Constant  relop===  const=1  OutDataTypeStr=boolean
  Compare To Constant off1 : simulink/Logic and Bit Operations/Compare To Constant  relop===  const=1  OutDataTypeStr=boolean
  Compare To Constant off2 : simulink/Logic and Bit Operations/Compare To Constant  relop===  const=32  OutDataTypeStr=boolean
  Compare To Constant on : simulink/Logic and Bit Operations/Compare To Constant  relop===  const=0  OutDataTypeStr=boolean
  Compare To Constant on1 : simulink/Logic and Bit Operations/Compare To Constant  relop===  const=0  OutDataTypeStr=boolean
  Compare To Constant on2 : simulink/Logic and Bit Operations/Compare To Constant  relop===  const=12  OutDataTypeStr=boolean
  Constant : Constant  Value=12
  Constant1 : Constant  Value=32
  Constant2 : Constant  Value=32
  Constant3 : Constant  Value=12
  Constant{4..7} (4 alike) : Constant  Value=0
  If : If  NumInputs=3  IfExpression=u1 > 0.5 & u3 >= u2  ElseIfExpressions=u1 > 0.5 & u3 < u2, u1 < -0.5 & u3 <= u2, u1 < -0.5 & u3 > u2
  If Action Subsystem : Subsystem  TreatAsAtomicUnit=on
  If Action Subsystem1 : Subsystem  TreatAsAtomicUnit=on
  If Action Subsystem10 : Subsystem  TreatAsAtomicUnit=on
  If Action Subsystem11 : Subsystem  TreatAsAtomicUnit=on
  If Action Subsystem12 : Subsystem  TreatAsAtomicUnit=on
  If Action Subsystem2 : Subsystem  TreatAsAtomicUnit=on
  If Action Subsystem3 : Subsystem  TreatAsAtomicUnit=on
  If Action Subsystem4 : Subsystem  TreatAsAtomicUnit=on
  If Action Subsystem5 : Subsystem  TreatAsAtomicUnit=on
  If Action Subsystem6 : Subsystem  TreatAsAtomicUnit=on
  If Action Subsystem7 : Subsystem  TreatAsAtomicUnit=on
  If Action Subsystem8 : Subsystem  TreatAsAtomicUnit=on
  If Action Subsystem9 : Subsystem  TreatAsAtomicUnit=on
  If1 : If  NumInputs=3  IfExpression=u1 > 0.5 & u3 < u2
  If2 : If  NumInputs=3  IfExpression=u1 < -0.5 & u3 > u2
  If3 : If  NumInputs=2  IfExpression=u1 < -0.5 & u2 > 0
  If4 : If  NumInputs=2  IfExpression=u1 > 0.5 & u2 > 0
  IsNaN : RelationalOperator  Operator=isNaN  OutDataTypeStr=boolean  RndMeth=Simplest
  Logical Operator low : Logic  AllPortsSameDT=off  OutDataTypeStr=boolean
  Logical Operator low1 : Logic  AllPortsSameDT=off  OutDataTypeStr=boolean
  Logical Operator low2 : Logic  AllPortsSameDT=off  OutDataTypeStr=boolean
  Logical Operator up : Logic  AllPortsSameDT=off  OutDataTypeStr=boolean
  Logical Operator up1 : Logic  AllPortsSameDT=off  OutDataTypeStr=boolean
  Logical Operator up2 : Logic  AllPortsSameDT=off  OutDataTypeStr=boolean
  Memory : Memory
  Memory1 : Memory
  Memory2 : Memory  InitialCondition=12
  Merge : Merge  Inputs=5
  Merge{1..4} (4 alike) : Merge
  Relational Operator dn : RelationalOperator  Operator=<  OutDataTypeStr=boolean  RndMeth=Simplest
  Relational Operator dn1 : RelationalOperator  Operator=<  OutDataTypeStr=boolean  RndMeth=Simplest
  Relational Operator dn2 : RelationalOperator  Operator=<  OutDataTypeStr=boolean  RndMeth=Simplest
  Relational Operator up : RelationalOperator  Operator=>  OutDataTypeStr=boolean  RndMeth=Simplest
  Relational Operator up1 : RelationalOperator  Operator=>  OutDataTypeStr=boolean  RndMeth=Simplest
  Relational Operator up2 : RelationalOperator  Operator=>  OutDataTypeStr=boolean  RndMeth=Simplest
  Switch{,1..5,8..10} (9 alike) : Switch  Criteria=u2 > Threshold
  off : Constant
  off1 : Constant
  off2 : Constant  Value=32
  on : Constant  Value=0
  on1 : Constant  Value=0
  on2 : Constant  Value=12
  on{3..6} (4 alike) : Constant  Value=0.1808
  R273 Heating : Outport
  R273 Cooling : Outport  Port=2
  R273 Setpoint Temperature : Outport  Port=3
  wires:
  Switch3/1 -> Memory/1, If4/2
  Memory/1 -> Compare To Constant on/1, Compare To Constant off/1, Switch4/3
  Memory1/1 -> Compare To Constant on1/1, Compare To Constant off1/1, Switch10/3
  on1/1 -> Switch9/1
  off/1 -> Switch4/1
  Relational Operator up1/1 -> Logical Operator low1/1
  Relational Operator dn1/1 -> Logical Operator up1/1
  Current Temperature/1 -> [tair]
  Compare To Constant off1/1 -> Logical Operator up1/2
  Compare To Constant on/1 -> Logical Operator low/2
  Upper Temperature Bound/1 -> [tup]
  Relational Operator up/1 -> Logical Operator up/1
  Compare To Constant on1/1 -> Logical Operator low1/2
  Logical Operator low1/1 -> Switch10/2
  on/1 -> Switch3/1
  Relational Operator dn/1 -> Logical Operator low/1
  Compare To Constant off/1 -> Logical Operator up/2
  Logical Operator up/1 -> Switch3/2
  Logical Operator low/1 -> Switch4/2
  Logical Operator up1/1 -> Switch9/2
  off1/1 -> Switch10/1
  Switch10/1 -> Switch9/3
  Switch4/1 -> Switch3/3
  Lower Temperature Bound/1 -> [tdn]
  Switch9/1 -> If3/2, Memory1/1
  Setpoint Override/1 -> IsNaN/1, [sp]
  [expr] -> Switch2/2
  Switch2/1 -> R273 Setpoint Temperature/1
  Compare To Constant off2/1 -> Logical Operator up2/2
  Logical Operator up2/1 -> Switch/2
  Memory2/1 -> Compare To Constant on2/1, Compare To Constant off2/1, Switch1/3
  on2/1 -> Switch/1
  Switch1/1 -> Switch/3
  [tup] -> Relational Operator up2/2
  [tdn] -> Relational Operator dn2/2
  Logical Operator low2/1 -> Switch1/2
  off2/1 -> Switch1/1
  Compare To Constant on2/1 -> Logical Operator low2/2
  Relational Operator up2/1 -> Logical Operator up2/1
  Relational Operator dn2/1 -> Logical Operator low2/1
  [expr] -> Switch5/2
  [expr] -> Switch8/2
  [tair] -> Relational Operator up/1
  [tair] -> Relational Operator dn/1
  [tair] -> Relational Operator dn1/1
  [tair] -> Relational Operator up1/1
  [tair] -> Relational Operator up2/1
  [tair] -> Relational Operator dn2/1
  [tdn] -> Relational Operator dn/2
  [tdn] -> Relational Operator dn1/2
  [tup] -> Relational Operator up/2
  [tup] -> Relational Operator up1/2
  AC mode/1 -> [ac]
  [ac] -> If/1
  [sp] -> If/2
  [tair] -> If Action Subsystem4/1(In1), If/3
  If/1 -> If Action Subsystem/Action
  Constant/1 -> If Action Subsystem/1(In1)
  If/3 -> If Action Subsystem1/Action
  If/2 -> If Action Subsystem2/Action
  Constant1/1 -> If Action Subsystem2/1(In1)
  If/4 -> If Action Subsystem3/Action
  Constant2/1 -> If Action Subsystem1/1(In1)
  Constant3/1 -> If Action Subsystem3/1(In1)
  If/5 -> If Action Subsystem4/Action
  If Action Subsystem/1(Out1) -> Merge/1
  If Action Subsystem2/1(Out1) -> Merge/2
  If Action Subsystem1/1(Out1) -> Merge/3
  If Action Subsystem3/1(Out1) -> Merge/4
  If Action Subsystem4/1(Out1) -> Merge/5
  [sp] -> If1/2
  on3/1 -> If Action Subsystem5/1(In1)
  [ac] -> If1/1
  If1/1 -> If Action Subsystem5/Action
  [tair] -> If1/3
  Merge1/1 -> Switch5/3
  If Action Subsystem5/1(Out1) -> Merge1/1
  If1/2 -> If Action Subsystem9/Action
  If Action Subsystem9/1(Out1) -> Merge1/2
  Constant5/1 -> If Action Subsystem9/1(In1)
  If2/2 -> If Action Subsystem7/Action
  If2/1 -> If Action Subsystem6/Action
  [ac] -> If2/1
  [sp] -> If2/2
  [tair] -> If2/3
  Constant4/1 -> If Action Subsystem7/1(In1)
  on4/1 -> If Action Subsystem6/1(In1)
  If Action Subsystem7/1(Out1) -> Merge2/2
  If Action Subsystem6/1(Out1) -> Merge2/1
  Merge2/1 -> Switch8/3
  Merge/1 -> Switch2/3
  Switch8/1 -> R273 Cooling/1
  If Action Subsystem8/1(Out1) -> Merge3/1
  If Action Subsystem10/1(Out1) -> Merge3/2
  Merge3/1 -> Switch8/1
  [ac] -> If3/1
  [ac] -> If4/1
  Switch5/1 -> R273 Heating/1
  Merge4/1 -> Switch5/1
  If3/1 -> If Action Subsystem8/Action
  If3/2 -> If Action Subsystem10/Action
  on5/1 -> If Action Subsystem8/1(In1)
  Constant6/1 -> If Action Subsystem10/1(In1)
  If4/2 -> If Action Subsystem11/Action
  Constant7/1 -> If Action Subsystem11/1(In1)
  on6/1 -> If Action Subsystem12/1(In1)
  If4/1 -> If Action Subsystem12/Action
  If Action Subsystem12/1(Out1) -> Merge4/1
  If Action Subsystem11/1(Out1) -> Merge4/2
  IsNaN/1 -> [expr]
  Switch/1 -> Switch2/1, Memory2/1

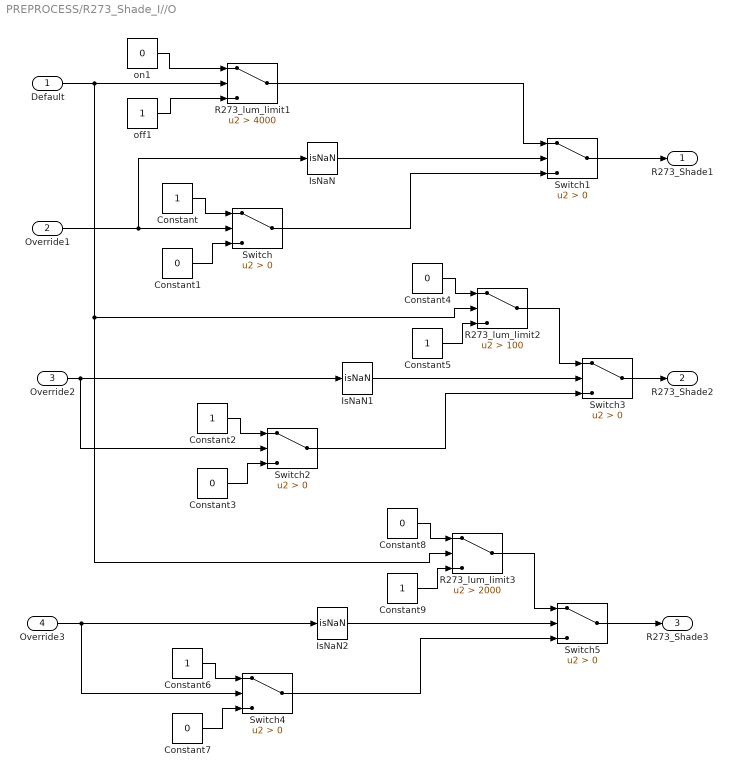
== system PREPROCESS/R273_Shade_I//O ==
  Default : Inport
  Override1 : Inport  Port=2
  Override2 : Inport  Port=3
  Override3 : Inport  Port=4
  Constant{,2,5..6,9} (5 alike) : Constant
  Constant{1,3..4,7..8} (5 alike) : Constant  Value=0
  IsNaN : RelationalOperator  Operator=isNaN  OutDataTypeStr=boolean  RndMeth=Simplest
  IsNaN1 : RelationalOperator  Operator=isNaN  OutDataTypeStr=boolean  RndMeth=Simplest
  IsNaN2 : RelationalOperator  Operator=isNaN  OutDataTypeStr=boolean  RndMeth=Simplest
  R273_lum_limit1 : Switch  Criteria=u2 > Threshold  Threshold=4000
  R273_lum_limit2 : Switch  Criteria=u2 > Threshold  Threshold=100
  R273_lum_limit3 : Switch  Criteria=u2 > Threshold  Threshold=2000
  Switch{,1..5} (6 alike) : Switch  Criteria=u2 > Threshold
  off1 : Constant
  on1 : Constant  Value=0
  R273_Shade1 : Outport
  R273_Shade2 : Outport  Port=2
  R273_Shade3 : Outport  Port=3
  wires:
  R273_lum_limit1/1 -> Switch1/1
  IsNaN/1 -> Switch1/2
  Switch1/1 -> R273_Shade1/1
  Constant1/1 -> Switch/3
  on1/1 -> R273_lum_limit1/1
  Constant/1 -> Switch/1
  Override1/1 -> IsNaN/1, Switch/2
  Default/1 -> R273_lum_limit3/2, R273_lum_limit2/2, R273_lum_limit1/2
  off1/1 -> R273_lum_limit1/3
  Switch/1 -> Switch1/3
  R273_lum_limit2/1 -> Switch3/1
  Constant3/1 -> Switch2/3
  Constant2/1 -> Switch2/1
  Switch2/1 -> Switch3/3
  Override2/1 -> Switch2/2, IsNaN1/1
  IsNaN1/1 -> Switch3/2
  Switch3/1 -> R273_Shade2/1
  Constant4/1 -> R273_lum_limit2/1
  Constant5/1 -> R273_lum_limit2/3
  Constant8/1 -> R273_lum_limit3/1
  Constant9/1 -> R273_lum_limit3/3
  Switch4/1 -> Switch5/3
  IsNaN2/1 -> Switch5/2
  Constant6/1 -> Switch4/1
  Constant7/1 -> Switch4/3
  Override3/1 -> IsNaN2/1, Switch4/2
  R273_lum_limit3/1 -> Switch5/1
  Switch5/1 -> R273_Shade3/1

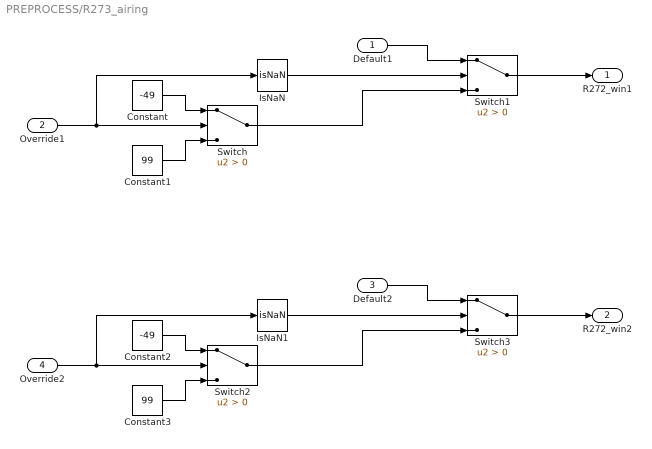
== system PREPROCESS/R273_airing ==
  Default1 : Inport
  Override1 : Inport  Port=2
  Default2 : Inport  Port=3
  Override2 : Inport  Port=4
  Constant : Constant  Value=-49
  Constant1 : Constant  Value=99
  Constant2 : Constant  Value=-49
  Constant3 : Constant  Value=99
  IsNaN : RelationalOperator  Operator=isNaN  OutDataTypeStr=boolean  RndMeth=Simplest
  IsNaN1 : RelationalOperator  Operator=isNaN  OutDataTypeStr=boolean  RndMeth=Simplest
  Switch{,1..3} (4 alike) : Switch  Criteria=u2 > Threshold
  R272_win1 : Outport
  R272_win2 : Outport  Port=2
  wires:
  Switch1/1 -> R272_win1/1
  IsNaN/1 -> Switch1/2
  Switch/1 -> Switch1/3
  Default1/1 -> Switch1/1
  Constant1/1 -> Switch/3
  Constant/1 -> Switch/1
  Override1/1 -> IsNaN/1, Switch/2
  Default2/1 -> Switch3/1
  Constant3/1 -> Switch2/3
  Switch2/1 -> Switch3/3
  Constant2/1 -> Switch2/1
  Override2/1 -> IsNaN1/1, Switch2/2
  Switch3/1 -> R272_win2/1
  IsNaN1/1 -> Switch3/2

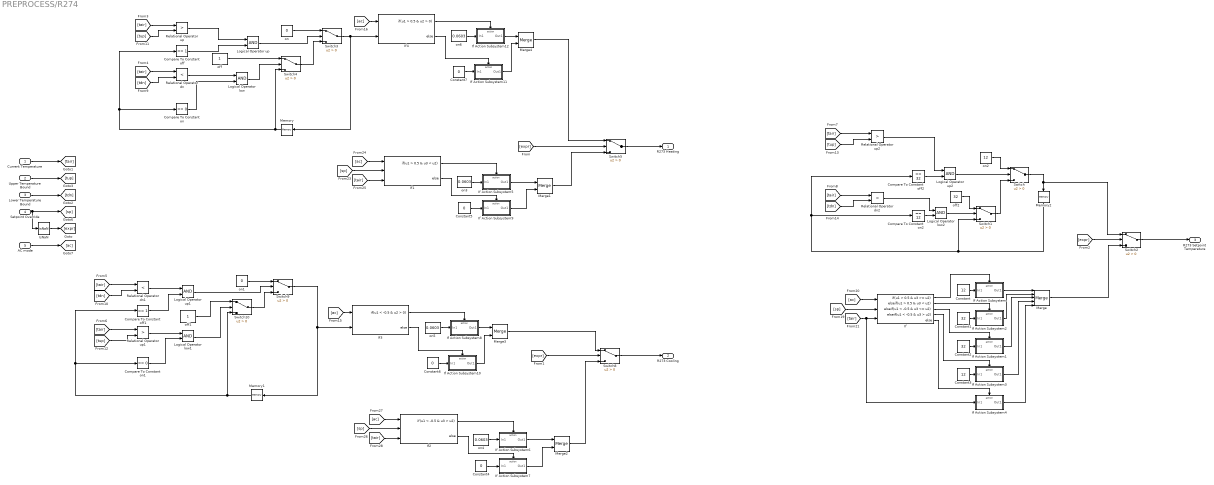
== system PREPROCESS/R274 ==
  Current Temperature : Inport
  Upper Temperature Bound : Inport  Port=2
  Lower Temperature Bound : Inport  Port=3
  Setpoint Override : Inport  Port=4
  AC mode : Inport  Port=5
  Compare To Constant off : simulink/Logic and Bit Operations/Compare To Constant  relop===  const=1  OutDataTypeStr=boolean
  Compare To Constant off1 : simulink/Logic and Bit Operations/Compare To Constant  relop===  const=1  OutDataTypeStr=boolean
  Compare To Constant off2 : simulink/Logic and Bit Operations/Compare To Constant  relop===  const=32  OutDataTypeStr=boolean
  Compare To Constant on : simulink/Logic and Bit Operations/Compare To Constant  relop===  const=0  OutDataTypeStr=boolean
  Compare To Constant on1 : simulink/Logic and Bit Operations/Compare To Constant  relop===  const=0  OutDataTypeStr=boolean
  Compare To Constant on2 : simulink/Logic and Bit Operations/Compare To Constant  relop===  const=12  OutDataTypeStr=boolean
  Constant : Constant  Value=12
  Constant1 : Constant  Value=32
  Constant2 : Constant  Value=32
  Constant3 : Constant  Value=12
  Constant{4..7} (4 alike) : Constant  Value=0
  If : If  NumInputs=3  IfExpression=u1 > 0.5 & u3 >= u2  ElseIfExpressions=u1 > 0.5 & u3 < u2, u1 < -0.5 & u3 <= u2, u1 < -0.5 & u3 > u2
  If Action Subsystem : Subsystem  TreatAsAtomicUnit=on
  If Action Subsystem1 : Subsystem  TreatAsAtomicUnit=on
  If Action Subsystem10 : Subsystem  TreatAsAtomicUnit=on
  If Action Subsystem11 : Subsystem  TreatAsAtomicUnit=on
  If Action Subsystem12 : Subsystem  TreatAsAtomicUnit=on
  If Action Subsystem2 : Subsystem  TreatAsAtomicUnit=on
  If Action Subsystem3 : Subsystem  TreatAsAtomicUnit=on
  If Action Subsystem4 : Subsystem  TreatAsAtomicUnit=on
  If Action Subsystem5 : Subsystem  TreatAsAtomicUnit=on
  If Action Subsystem6 : Subsystem  TreatAsAtomicUnit=on
  If Action Subsystem7 : Subsystem  TreatAsAtomicUnit=on
  If Action Subsystem8 : Subsystem  TreatAsAtomicUnit=on
  If Action Subsystem9 : Subsystem  TreatAsAtomicUnit=on
  If1 : If  NumInputs=3  IfExpression=u1 > 0.5 & u3 < u2
  If2 : If  NumInputs=3  IfExpression=u1 < -0.5 & u3 > u2
  If3 : If  NumInputs=2  IfExpression=u1 < -0.5 & u2 > 0
  If4 : If  NumInputs=2  IfExpression=u1 > 0.5 & u2 > 0
  IsNaN : RelationalOperator  Operator=isNaN  OutDataTypeStr=boolean  RndMeth=Simplest
  Logical Operator low : Logic  AllPortsSameDT=off  OutDataTypeStr=boolean
  Logical Operator low1 : Logic  AllPortsSameDT=off  OutDataTypeStr=boolean
  Logical Operator low2 : Logic  AllPortsSameDT=off  OutDataTypeStr=boolean
  Logical Operator up : Logic  AllPortsSameDT=off  OutDataTypeStr=boolean
  Logical Operator up1 : Logic  AllPortsSameDT=off  OutDataTypeStr=boolean
  Logical Operator up2 : Logic  AllPortsSameDT=off  OutDataTypeStr=boolean
  Memory : Memory
  Memory1 : Memory
  Memory2 : Memory  InitialCondition=12
  Merge : Merge  Inputs=5
  Merge{1..4} (4 alike) : Merge
  Relational Operator dn : RelationalOperator  Operator=<  OutDataTypeStr=boolean  RndMeth=Simplest
  Relational Operator dn1 : RelationalOperator  Operator=<  OutDataTypeStr=boolean  RndMeth=Simplest
  Relational Operator dn2 : RelationalOperator  Operator=<  OutDataTypeStr=boolean  RndMeth=Simplest
  Relational Operator up : RelationalOperator  Operator=>  OutDataTypeStr=boolean  RndMeth=Simplest
  Relational Operator up1 : RelationalOperator  Operator=>  OutDataTypeStr=boolean  RndMeth=Simplest
  Relational Operator up2 : RelationalOperator  Operator=>  OutDataTypeStr=boolean  RndMeth=Simplest
  Switch{,1..5,8..10} (9 alike) : Switch  Criteria=u2 > Threshold
  off : Constant
  off1 : Constant
  off2 : Constant  Value=32
  on : Constant  Value=0
  on1 : Constant  Value=0
  on2 : Constant  Value=12
  on{3..6} (4 alike) : Constant  Value=0.0603
  R273 Heating : Outport
  R273 Cooling : Outport  Port=2
  R273 Setpoint Temperature : Outport  Port=3
  wires:
  If3/1 -> If Action Subsystem8/Action
  If2/1 -> If Action Subsystem6/Action
  If Action Subsystem3/1(Out1) -> Merge/4
  [tair] -> If Action Subsystem4/1(In1), If/3
  [sp] -> If/2
  Relational Operator dn/1 -> Logical Operator low/1
  [tup] -> Relational Operator up/2
  Constant7/1 -> If Action Subsystem11/1(In1)
  [expr] -> Switch5/2
  If1/2 -> If Action Subsystem9/Action
  Merge2/1 -> Switch8/3
  on6/1 -> If Action Subsystem12/1(In1)
  If Action Subsystem10/1(Out1) -> Merge3/2
  [tair] -> If1/3
  on2/1 -> Switch/1
  IsNaN/1 -> [expr]
  If4/2 -> If Action Subsystem11/Action
  If Action Subsystem11/1(Out1) -> Merge4/2
  If4/1 -> If Action Subsystem12/Action
  Constant4/1 -> If Action Subsystem7/1(In1)
  Switch8/1 -> R273 Cooling/1
  [sp] -> If1/2
  If Action Subsystem8/1(Out1) -> Merge3/1
  on4/1 -> If Action Subsystem6/1(In1)
  If/5 -> If Action Subsystem4/Action
  [ac] -> If4/1
  Switch4/1 -> Switch3/3
  Switch9/1 -> If3/2, Memory1/1
  [sp] -> If2/2
  If3/2 -> If Action Subsystem10/Action
  Switch5/1 -> R273 Heating/1
  Constant6/1 -> If Action Subsystem10/1(In1)
  Relational Operator up2/1 -> Logical Operator up2/1
  on5/1 -> If Action Subsystem8/1(In1)
  Compare To Constant on/1 -> Logical Operator low/2
  Lower Temperature Bound/1 -> [tdn]
  Constant2/1 -> If Action Subsystem1/1(In1)
  If Action Subsystem4/1(Out1) -> Merge/5
  Compare To Constant off/1 -> Logical Operator up/2
  Merge4/1 -> Switch5/1
  If1/1 -> If Action Subsystem5/Action
  [ac] -> If3/1
  Merge3/1 -> Switch8/1
  AC mode/1 -> [ac]
  Logical Operator up/1 -> Switch3/2
  If Action Subsystem6/1(Out1) -> Merge2/1
  Memory/1 -> Compare To Constant on/1, Compare To Constant off/1, Switch4/3
  If/2 -> If Action Subsystem2/Action
  on3/1 -> If Action Subsystem5/1(In1)
  Merge1/1 -> Switch5/3
  If Action Subsystem9/1(Out1) -> Merge1/2
  If Action Subsystem/1(Out1) -> Merge/1
  Logical Operator low1/1 -> Switch10/2
  If/3 -> If Action Subsystem1/Action
  [tair] -> Relational Operator up2/1
  off1/1 -> Switch10/1
  [ac] -> If2/1
  Setpoint Override/1 -> IsNaN/1, [sp]
  Relational Operator dn2/1 -> Logical Operator low2/1
  If Action Subsystem12/1(Out1) -> Merge4/1
  Compare To Constant off2/1 -> Logical Operator up2/2
  Switch10/1 -> Switch9/3
  [ac] -> If/1
  Relational Operator up1/1 -> Logical Operator low1/1
  Relational Operator dn1/1 -> Logical Operator up1/1
  [tup] -> Relational Operator up1/2
  off/1 -> Switch4/1
  [expr] -> Switch2/2
  [expr] -> Switch8/2
  Constant/1 -> If Action Subsystem/1(In1)
  [tair] -> Relational Operator dn1/1
  [tair] -> Relational Operator up1/1
  [tdn] -> Relational Operator dn2/2
  Constant5/1 -> If Action Subsystem9/1(In1)
  If Action Subsystem7/1(Out1) -> Merge2/2
  Logical Operator low2/1 -> Switch1/2
  [tup] -> Relational Operator up2/2
  Merge/1 -> Switch2/3
  on/1 -> Switch3/1
  Constant3/1 -> If Action Subsystem3/1(In1)
  If/4 -> If Action Subsystem3/Action
  Logical Operator low/1 -> Switch4/2
  [tdn] -> Relational Operator dn1/2
  on1/1 -> Switch9/1
  Logical Operator up1/1 -> Switch9/2
  Compare To Constant off1/1 -> Logical Operator up1/2
  Relational Operator up/1 -> Logical Operator up/1
  Logical Operator up2/1 -> Switch/2
  Current Temperature/1 -> [tair]
  [tair] -> Relational Operator up/1
  [tair] -> Relational Operator dn/1
  If Action Subsystem1/1(Out1) -> Merge/3
  Compare To Constant on2/1 -> Logical Operator low2/2
  [tair] -> If2/3
  Switch3/1 -> Memory/1, If4/2
  Switch/1 -> Switch2/1, Memory2/1
  Constant1/1 -> If Action Subsystem2/1(In1)
  If Action Subsystem5/1(Out1) -> Merge1/1
  [tdn] -> Relational Operator dn/2
  Switch1/1 -> Switch/3
  off2/1 -> Switch1/1
  Memory1/1 -> Compare To Constant on1/1, Compare To Constant off1/1, Switch10/3
  Memory2/1 -> Compare To Constant on2/1, Compare To Constant off2/1, Switch1/3
  Upper Temperature Bound/1 -> [tup]
  Compare To Constant on1/1 -> Logical Operator low1/2
  [tair] -> Relational Operator dn2/1
  If/1 -> If Action Subsystem/Action
  [ac] -> If1/1
  If Action Subsystem2/1(Out1) -> Merge/2
  If2/2 -> If Action Subsystem7/Action
  Switch2/1 -> R273 Setpoint Temperature/1

== system PREPROCESS/R274_Shade_I//O ==
  Default : Inport
  Override : Inport  Port=2
  Constant : Constant
  Constant1 : Constant  Value=0
  IsNaN : RelationalOperator  Operator=isNaN  OutDataTypeStr=boolean  RndMeth=Simplest
  R272_lum_limit : Switch  Criteria=u2 > Threshold  Threshold=50
  Switch : Switch  Criteria=u2 > Threshold
  Switch1 : Switch  Criteria=u2 > Threshold
  off1 : Constant
  on1 : Constant  Value=0
  R274_Shade : Outport
  wires:
  R272_lum_limit/1 -> Switch1/1
  IsNaN/1 -> Switch1/2
  Switch1/1 -> R274_Shade/1
  Constant1/1 -> Switch/3
  on1/1 -> R272_lum_limit/1
  Constant/1 -> Switch/1
  Override/1 -> IsNaN/1, Switch/2
  Default/1 -> R272_lum_limit/2
  off1/1 -> R272_lum_limit/3
  Switch/1 -> Switch1/3

== system PREPROCESS/R274_airing ==
  Default : Inport
  Override : Inport  Port=2
  Constant : Constant  Value=-49
  Constant1 : Constant  Value=99
  IsNaN : RelationalOperator  Operator=isNaN  OutDataTypeStr=boolean  RndMeth=Simplest
  Switch : Switch  Criteria=u2 > Threshold
  Switch1 : Switch  Criteria=u2 > Threshold
  R274_win : Outport
  wires:
  Constant1/1 -> Switch/3
  Switch/1 -> Switch1/3
  Constant/1 -> Switch/1
  Switch1/1 -> R274_win/1
  IsNaN/1 -> Switch1/2
  Override/1 -> Switch/2
  Default/1 -> Switch1/1
